simulink model "Squelette_DSPBuilder_FrameGenerator"  (R2016a)
settings: Solver=FixedStepDiscrete  StartTime=0.0  StopTime=2e-3  RelTol=1e-3
InitFcn:
  | %% DSPBuilder Start
  | alt_dspbuilder_update_model(bdroot)
  | %% DSPBuilder End
libraries: allblocks_alteradspbuilder2 x55
settings Model: Creator=rhev2401  LastModifiedBy=dufd2703
settings DataIOCC: LimitDataPoints=on  SaveFormat=Array  SignalLoggingSaveFormat=ModelDataLogs
settings DebuggingCC: SolverPrmCheckMsg=warning  MultiTaskDSMMsg=warning  MultiTaskCondExecSysMsg=none
settings HardwareCC: ProdBitPerPointer=32  ProdLargestAtomicFloat=None  ProdIntDivRoundTo=Undefined  ProdEndianess=Unspecified  ProdWordSize=32  ProdHWDeviceType=32-bit Generic
settings ModelReferenceCC: PropagateSignalLabelsOutOfModel=off
settings ConfigComp: CovModelRefEnable=Off  CovSFcnEnable=off

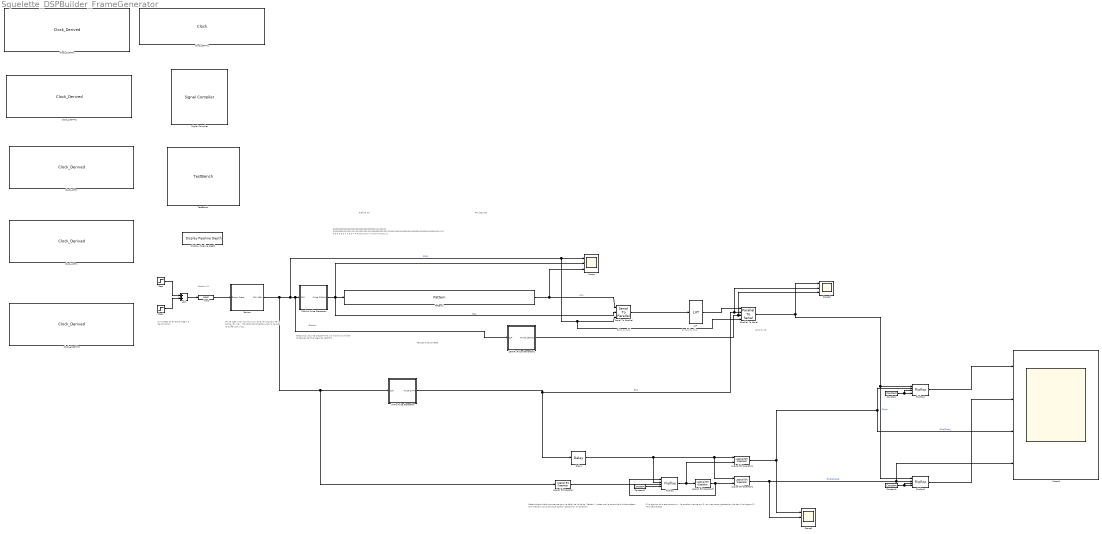
== system Squelette_DSPBuilder_FrameGenerator ==
  note: Simulates an event to begin a transmission
  note: Payload 80
  note: Prefixe 40
  note: 0000000000000000000000000000000011100101 10010000111011111111001101110100000101101110010100110001010100001010000110000110
      | 0 0 0 0 0 0 0 0 7 A 9 0 7 F F C E 2 8 6 7 A C 8 A 0 5 8 1 6
  note: Bouton 01
  note: On se crée une impulsion qui dure la longueur de la trame.
      |
      | En vrai, il faudrait transmettre jusqu'à ce que le buffer soit vide...
  note: Paquet à transmettre
  note: Bitclock
  note: Notez que, pour ce programme, on a choisi d'utiliser la fréquence d'horloge de 100MHz.
  note: Bit to symbol
  note: Symbol to chip
  note: Chip to I/Q
  note: Si le dernier chip est rentré sur I, le prochain rentre sur Q, et vice-versa; génération de deux horloges d'1 MHz déphasées
  note: Cette boîte à délai compense pour le délai de la boîte "Pattern" (notez que la sortie de la boîte pattern commence 1 coup de clock après l'apparition du Enable)
  250kHz Pulse Generator : Subsystem
  250kHz Pulse Generator1 : Subsystem
  2MHz Pulse Generator : Subsystem
  Add : Sum
  Bouton : Subsystem
  Clock_100MHz : allblocks_alteradspbuilder2/Clock_Derived  ClockNumerator=1  ClockDenominator=2  ResetLatency=0  ResetRegisterCascadeDepth=0  SimulationStartCycle=5  PhaseOffset=0  Reset=aclr_100MHz  ResetType=Active Low  Export=off
  Clock_125MHz : allblocks_alteradspbuilder2/Clock_Derived  ClockNumerator=10  ClockDenominator=25  ResetLatency=0  ResetRegisterCascadeDepth=0  SimulationStartCycle=5  PhaseOffset=0  Reset=aclr_125MHz  ResetType=Active Low  Export=off
  Clock_1MHz : allblocks_alteradspbuilder2/Clock_Derived  ClockNumerator=50  ClockDenominator=1  ResetLatency=0  ResetRegisterCascadeDepth=0  SimulationStartCycle=5  PhaseOffset=0  Reset=aclr_1MHz  ResetType=Active Low  Export=off
  Clock_2MHz : allblocks_alteradspbuilder2/Clock_Derived  ClockNumerator=25  ClockDenominator=1  ResetLatency=0  ResetRegisterCascadeDepth=0  SimulationStartCycle=5  PhaseOffset=0  Reset=aclr_2MHz  ResetType=Active Low  Export=off
  Clock_50MHz : allblocks_alteradspbuilder2/Clock  ClockPeriod=20  ClockPeriodUnit=ns  SampleTime=20e-9  ResetLatency=0  ResetRegisterCascadeDepth=0  SimulationStartCycle=5  PhaseOffset=0  Reset=aclr  ResetType=Active Low  Export=off
  Clock_62p5MHz : allblocks_alteradspbuilder2/Clock_Derived  ClockNumerator=800  ClockDenominator=1  ResetLatency=0  ResetRegisterCascadeDepth=0  SimulationStartCycle=5  PhaseOffset=0  Reset=aclr_62p5MHz  ResetType=Active Low  Export=off
  Constant : allblocks_alteradspbuilder2/Constant  mask_cst=1  BusType=Signed Integer  bwl=8  bwr=0  roundMode=Truncate  satMode=Wrap  SpecifyClock=off  allowFloatingPointOverride=on  logOutputs=off  logFile=U:\projet-s6\DSP builder\Squelette_FrameGenerator\tb_Squelette_DSPBuilder_FrameGenerator\Squelette%5FDSPBuilder%5FFrameGenerator_Constant.fixedpointlog
  Constant1 : allblocks_alteradspbuilder2/Constant  mask_cst=1  BusType=Signed Integer  bwl=8  bwr=0  roundMode=Truncate  satMode=Wrap  SpecifyClock=off  allowFloatingPointOverride=on  logOutputs=off  logFile=U:\projet-s6\DSP builder\Squelette_FrameGenerator\tb_Squelette_DSPBuilder_FrameGenerator\Squelette%5FDSPBuilder%5FFrameGenerator_Constant1.fixedpointlog
  Constant2 : allblocks_alteradspbuilder2/Constant  mask_cst=1  BusType=Signed Integer  bwl=8  bwr=0  roundMode=Truncate  satMode=Wrap  SpecifyClock=off  allowFloatingPointOverride=on  logOutputs=off  logFile=U:\projet-s6\DSP builder\Squelette_FrameGenerator\tb_Squelette_DSPBuilder_FrameGenerator\Squelette%5FDSPBuilder%5FFrameGenerator_Constant2.fixedpointlog
  Delay : allblocks_alteradspbuilder2/Delay  pipeline=1  pipeline_display=1  ClockPhase=1  use_ena=off  use_sclr=off  allowFloatingPointOverride=on  logOutputs=off  logFile=U:\projet-s6\DSP builder\Squelette_FrameGenerator\tb_Squelette_DSPBuilder_FrameGenerator\Squelette%5FDSPBuilder%5FFrameGenerator_Delay.fixedpointlog  use_init=off  reset_value=1
  Display Pipeline Depth : allblocks_alteradspbuilder2/Display Pipeline Depth  DisplayLatencyOnBlocks=on
  Flipflop : allblocks_alteradspbuilder2/Flipflop  mode=DFFE  BusType=Single Bit  bwl=2  bwr=2  pipeline_display=1
  Flipflop1 : allblocks_alteradspbuilder2/Flipflop  mode=DFFE  BusType=Single Bit  bwl=2  bwr=2  pipeline_display=1
  Flipflop2 : allblocks_alteradspbuilder2/Flipflop  mode=DFFE  BusType=Single Bit  bwl=2  bwr=2  pipeline_display=1
  Input : allblocks_alteradspbuilder2/Input  iofile=U:\projet-s6\DSP builder\Squelette_FrameGenerator\tb_Squelette_DSPBuilder_FrameGenerator\Squelette%5FDSPBuilder%5FFrameGenerator_Input.salt  BusType=Single Bit  bwl=1  bwr=0  SpecifyClock=on  clock=Clock_100MHz  PORTTYPE=Input  externalType=Inferred  allowFloatingPointOverride=on  logOutputs=off
  LUT : allblocks_alteradspbuilder2/LUT  addr_width=4  BusType=Unsigned Integer  bwl=32  bwr=0  init_array=chips_lut  allowFloatingPointOverride=on  logOutputs=off  logFile=U:\projet-s6\DSP builder\Squelette_FrameGenerator\tb_Squelette_DSPBuilder_FrameGenerator\Squelette%5FDSPBuilder%5FFrameGenerator_LUT.fixedpointlog  use_ena=off  reg_data=off  use_lpm=on  reg_addr=on  ram_type=AUTO  pipeline_display=1
  Logical Bit Operator : allblocks_alteradspbuilder2/Logical Bit Operator  LogicalOperator=NOT  user_inputs=2  pipeline_display=0
  Logical Bit Operator1 : allblocks_alteradspbuilder2/Logical Bit Operator  LogicalOperator=AND  user_inputs=2  pipeline_display=0
  Logical Bit Operator2 : allblocks_alteradspbuilder2/Logical Bit Operator  LogicalOperator=AND  user_inputs=2  pipeline_display=0
  Logical Bit Operator3 : allblocks_alteradspbuilder2/Logical Bit Operator  LogicalOperator=NOT  user_inputs=2  pipeline_display=0
  Parallel To Serial : allblocks_alteradspbuilder2/Parallel To Serial  BusType=Unsigned Integer  bwl=32  bwr=0  msbfirsttext=MSB First  msbfirst=1  repeatlastbit=off  use_ena=on  use_sclr=on
  Pattern1 : allblocks_alteradspbuilder2/Pattern  Sequence=<binary blob, 120 chars, not shown>  SpecifyClock=off  clock=Clock_250kHz  use_ena=on  use_sclr=off
  Scope : Scope  NumInputPorts=3
  Scope1 : Scope  NumInputPorts=4
  Scope2 : Scope  NumInputPorts=3
  Scope3 : Scope  NumInputPorts=3
  Serial To Parallel : allblocks_alteradspbuilder2/Serial To Parallel  BusType=Unsigned Integer  bwl=4  bwr=0  msbfirsttext=MSB First  msbfirst=1  use_ena=on  use_sclr=on
  Signal Compiler : allblocks_alteradspbuilder2/Signal Compiler  DeviceFamily=Cyclone V  DeviceName=AUTO  DisableEarlyHDLGeneration=off  EnableSignalTap=off  SignalTapDepth=128  UseBoardBlock=off  StpUseDefaultClock=on  StpClock=Clock_50MHz  ExportDir=C:\Users\pivd2501\Documents  MAX10_ProgrammingMode=Internal Flash (SDM) Single Boot
  Step : Step  Time=100e-6  Before=1  After=0  SampleTime=1/100e06  VectorParams1D=off
  Step1 : Step  Time=200e-6  SampleTime=1/100e06  VectorParams1D=off
  TestBench : allblocks_alteradspbuilder2/TestBench  enable=on  advancedMode=on  modelSimGui=on  maxDisplayErrors=1000  mismatchErrorLevel=Error  simdatafile=U:\projet-s6\DSP builder\Squelette_FrameGenerator\tb_Squelette_DSPBuilder_FrameGenerator\Squelette_DSPBuilder_FrameGenerator.simdata.tcl
  wires:
  Add/1 -> Input/1
  Step1/1 -> Add/2
  Step/1 -> Add/1
  250kHz Pulse Generator/1(Pulse 250kHz) -> Serial To Parallel/2, Pattern1/1, Scope/2  "ENA"
  Pattern1/1 -> Serial To Parallel/1, Scope/3  "ATA"
  Input/1 -> Bouton/1(Button Press)
  Serial To Parallel/1 -> LUT/1
  LUT/1 -> Parallel To Serial/1
  2MHz Pulse Generator/1(Pulse 2MHz) -> Scope3/2, Parallel To Serial/2, Delay/1  "ENA"
  Parallel To Serial/1 -> Flipflop1/1, Flipflop2/1, Scope3/1  "Chips"
  Bouton/1(CLR 480u) -> Logical Bit Operator/1, 2MHz Pulse Generator/1(CLR), 250kHz Pulse Generator1/1(CLR), 250kHz Pulse Generator/1(CLR), Parallel To Serial/4, Serial To Parallel/3, Scope/1  "SCLR"
  Flipflop/1 -> Logical Bit Operator1/2, Logical Bit Operator3/1
  Logical Bit Operator3/1 -> Flipflop/1, Logical Bit Operator2/2
  Logical Bit Operator1/1 -> Scope2/1, Scope1/3, Flipflop1/2  "ChipClock_I"
  Constant/1 -> Flipflop1/4, Flipflop1/3
  Constant1/1 -> Flipflop2/3, Flipflop2/4
  Logical Bit Operator2/1 -> Scope2/2, Scope1/4, Flipflop2/2  "ChipClock_Q"
  Logical Bit Operator/1 -> Flipflop/3
  Constant2/1 -> Flipflop/4
  Delay/1 -> Flipflop/2, Logical Bit Operator2/1, Logical Bit Operator1/1
  Flipflop2/1 -> Scope1/2
  Flipflop1/1 -> Scope1/1
  250kHz Pulse Generator1/1(Pulse 250kHz) -> Scope3/3, Parallel To Serial/3

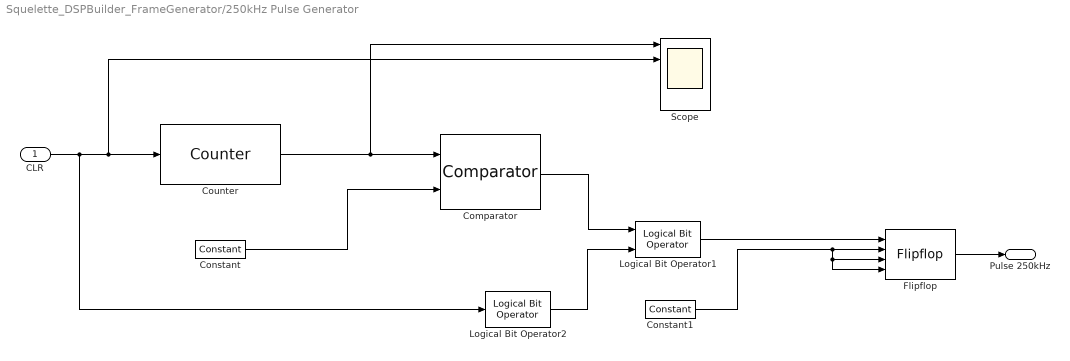
== system Squelette_DSPBuilder_FrameGenerator/250kHz Pulse Generator ==
  CLR : Inport
  Comparator : allblocks_alteradspbuilder2/Comparator  direction=a == b  pipeline_display=0  allowFloatingPointOverride=on  logOutputs=off  logFile=U:\projet-s6\DSP builder\Squelette_FrameGenerator\tb_Squelette_DSPBuilder_FrameGenerator\Squelette%5FDSPBuilder%5FFrameGenerator_250kHz+Pulse+Generator_Comparator.fixedpointlog
  Constant : allblocks_alteradspbuilder2/Constant  mask_cst=0  BusType=Unsigned Integer  bwl=1  bwr=0  roundMode=Truncate  satMode=Wrap  SpecifyClock=off  allowFloatingPointOverride=on  logOutputs=off  logFile=U:\projet-s6\DSP builder\Squelette_FrameGenerator\tb_Squelette_DSPBuilder_FrameGenerator\Squelette%5FDSPBuilder%5FFrameGenerator_250kHz+Pulse+Generator_Constant.fixedpointlog
  Constant1 : allblocks_alteradspbuilder2/Constant  mask_cst=1  BusType=Unsigned Integer  bwl=1  bwr=0  roundMode=Truncate  satMode=Wrap  SpecifyClock=off  allowFloatingPointOverride=on  logOutputs=off  logFile=U:\projet-s6\DSP builder\Squelette_FrameGenerator\tb_Squelette_DSPBuilder_FrameGenerator\Squelette%5FDSPBuilder%5FFrameGenerator_250kHz+Pulse+Generator_Constant1.fixedpointlog
  Counter : allblocks_alteradspbuilder2/Counter  BusType=Unsigned Integer  bwl=10  bwr=0  use_modulo=on  modulo=400  SpecifyClock=off  direction=Increment  use_sload=off  use_sset=off  svalue=1  use_clk_ena=off  use_ena=off  use_sclr=on  pipeline_display=1
  Flipflop : allblocks_alteradspbuilder2/Flipflop  mode=DFFE  BusType=Single Bit  bwl=2  bwr=2  pipeline_display=1
  Logical Bit Operator1 : allblocks_alteradspbuilder2/Logical Bit Operator  LogicalOperator=AND  user_inputs=2  pipeline_display=0
  Logical Bit Operator2 : allblocks_alteradspbuilder2/Logical Bit Operator  LogicalOperator=NOT  user_inputs=2  pipeline_display=0
  Scope : Scope  NumInputPorts=5
  Pulse 250kHz : Outport
  wires:
  Counter/1 -> Scope/1, Comparator/1
  Constant/1 -> Comparator/2
  CLR/1 -> Logical Bit Operator2/1, Scope/2, Counter/1
  Logical Bit Operator2/1 -> Logical Bit Operator1/2
  Comparator/1 -> Logical Bit Operator1/1
  Flipflop/1 -> Pulse 250kHz/1
  Logical Bit Operator1/1 -> Flipflop/1
  Constant1/1 -> Flipflop/4, Flipflop/3, Flipflop/2

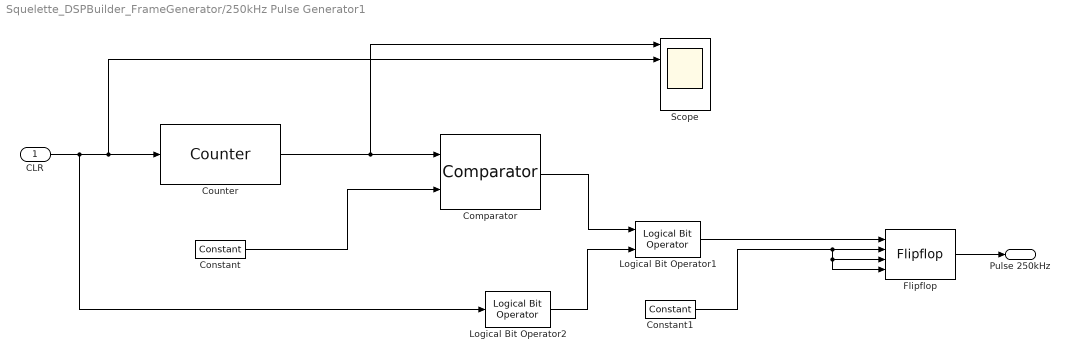
== system Squelette_DSPBuilder_FrameGenerator/250kHz Pulse Generator1 ==
  CLR : Inport
  Comparator : allblocks_alteradspbuilder2/Comparator  direction=a == b  pipeline_display=0  allowFloatingPointOverride=on  logOutputs=off  logFile=U:\projet-s6\DSP builder\Squelette_FrameGenerator\tb_Squelette_DSPBuilder_FrameGenerator\Squelette%5FDSPBuilder%5FFrameGenerator_250kHz+Pulse+Generator1_Comparator.fixedpointlog
  Constant : allblocks_alteradspbuilder2/Constant  mask_cst=0  BusType=Unsigned Integer  bwl=1  bwr=0  roundMode=Truncate  satMode=Wrap  SpecifyClock=off  allowFloatingPointOverride=on  logOutputs=off  logFile=U:\projet-s6\DSP builder\Squelette_FrameGenerator\tb_Squelette_DSPBuilder_FrameGenerator\Squelette%5FDSPBuilder%5FFrameGenerator_250kHz+Pulse+Generator1_Constant.fixedpointlog
  Constant1 : allblocks_alteradspbuilder2/Constant  mask_cst=1  BusType=Unsigned Integer  bwl=1  bwr=0  roundMode=Truncate  satMode=Wrap  SpecifyClock=off  allowFloatingPointOverride=on  logOutputs=off  logFile=U:\projet-s6\DSP builder\Squelette_FrameGenerator\tb_Squelette_DSPBuilder_FrameGenerator\Squelette%5FDSPBuilder%5FFrameGenerator_250kHz+Pulse+Generator1_Constant1.fixedpointlog
  Counter : allblocks_alteradspbuilder2/Counter  BusType=Unsigned Integer  bwl=12  bwr=0  use_modulo=on  modulo=1600  SpecifyClock=off  direction=Increment  use_sload=off  use_sset=off  svalue=1  use_clk_ena=off  use_ena=off  use_sclr=on  pipeline_display=1
  Flipflop : allblocks_alteradspbuilder2/Flipflop  mode=DFFE  BusType=Single Bit  bwl=2  bwr=2  pipeline_display=1
  Logical Bit Operator1 : allblocks_alteradspbuilder2/Logical Bit Operator  LogicalOperator=AND  user_inputs=2  pipeline_display=0
  Logical Bit Operator2 : allblocks_alteradspbuilder2/Logical Bit Operator  LogicalOperator=NOT  user_inputs=2  pipeline_display=0
  Scope : Scope  NumInputPorts=5
  Pulse 250kHz : Outport
  wires:
  Constant1/1 -> Flipflop/2, Flipflop/3, Flipflop/4
  Logical Bit Operator1/1 -> Flipflop/1
  Flipflop/1 -> Pulse 250kHz/1
  Comparator/1 -> Logical Bit Operator1/1
  Logical Bit Operator2/1 -> Logical Bit Operator1/2
  CLR/1 -> Counter/1, Scope/2, Logical Bit Operator2/1
  Constant/1 -> Comparator/2
  Counter/1 -> Comparator/1, Scope/1

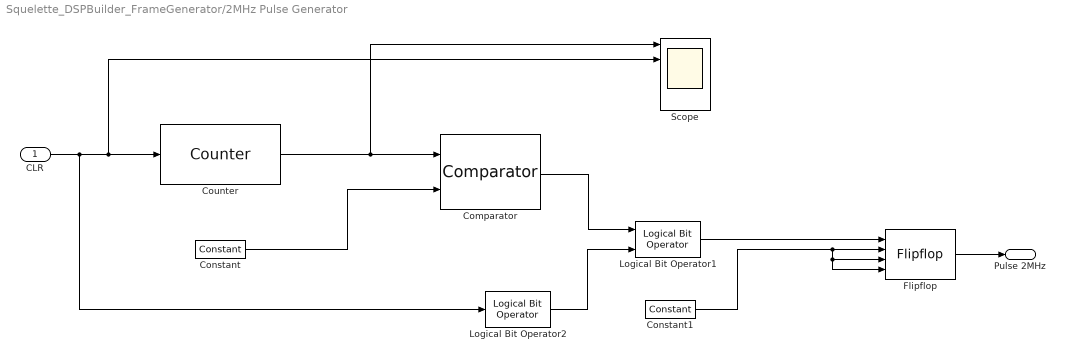
== system Squelette_DSPBuilder_FrameGenerator/2MHz Pulse Generator ==
  CLR : Inport
  Comparator : allblocks_alteradspbuilder2/Comparator  direction=a == b  pipeline_display=0  allowFloatingPointOverride=on  logOutputs=off  logFile=U:\projet-s6\DSP builder\Squelette_FrameGenerator\tb_Squelette_DSPBuilder_FrameGenerator\Squelette%5FDSPBuilder%5FFrameGenerator_2MHz+Pulse+Generator_Comparator.fixedpointlog
  Constant : allblocks_alteradspbuilder2/Constant  mask_cst=0  BusType=Unsigned Integer  bwl=1  bwr=0  roundMode=Truncate  satMode=Wrap  SpecifyClock=off  allowFloatingPointOverride=on  logOutputs=off  logFile=U:\projet-s6\DSP builder\Squelette_FrameGenerator\tb_Squelette_DSPBuilder_FrameGenerator\Squelette%5FDSPBuilder%5FFrameGenerator_2MHz+Pulse+Generator_Constant.fixedpointlog
  Constant1 : allblocks_alteradspbuilder2/Constant  mask_cst=1  BusType=Unsigned Integer  bwl=1  bwr=0  roundMode=Truncate  satMode=Wrap  SpecifyClock=off  allowFloatingPointOverride=on  logOutputs=off  logFile=U:\projet-s6\DSP builder\Squelette_FrameGenerator\tb_Squelette_DSPBuilder_FrameGenerator\Squelette%5FDSPBuilder%5FFrameGenerator_2MHz+Pulse+Generator_Constant1.fixedpointlog
  Counter : allblocks_alteradspbuilder2/Counter  BusType=Unsigned Integer  bwl=10  bwr=0  use_modulo=on  modulo=50  SpecifyClock=off  direction=Increment  use_sload=off  use_sset=off  svalue=1  use_clk_ena=off  use_ena=off  use_sclr=on  pipeline_display=1
  Flipflop : allblocks_alteradspbuilder2/Flipflop  mode=DFFE  BusType=Single Bit  bwl=2  bwr=2  pipeline_display=1
  Logical Bit Operator1 : allblocks_alteradspbuilder2/Logical Bit Operator  LogicalOperator=AND  user_inputs=2  pipeline_display=0
  Logical Bit Operator2 : allblocks_alteradspbuilder2/Logical Bit Operator  LogicalOperator=NOT  user_inputs=2  pipeline_display=0
  Scope : Scope  NumInputPorts=5
  Pulse 2MHz : Outport
  wires:
  Counter/1 -> Scope/1, Comparator/1
  Constant/1 -> Comparator/2
  CLR/1 -> Logical Bit Operator2/1, Scope/2, Counter/1
  Logical Bit Operator2/1 -> Logical Bit Operator1/2
  Comparator/1 -> Logical Bit Operator1/1
  Flipflop/1 -> Pulse 2MHz/1
  Logical Bit Operator1/1 -> Flipflop/1
  Constant1/1 -> Flipflop/4, Flipflop/3, Flipflop/2

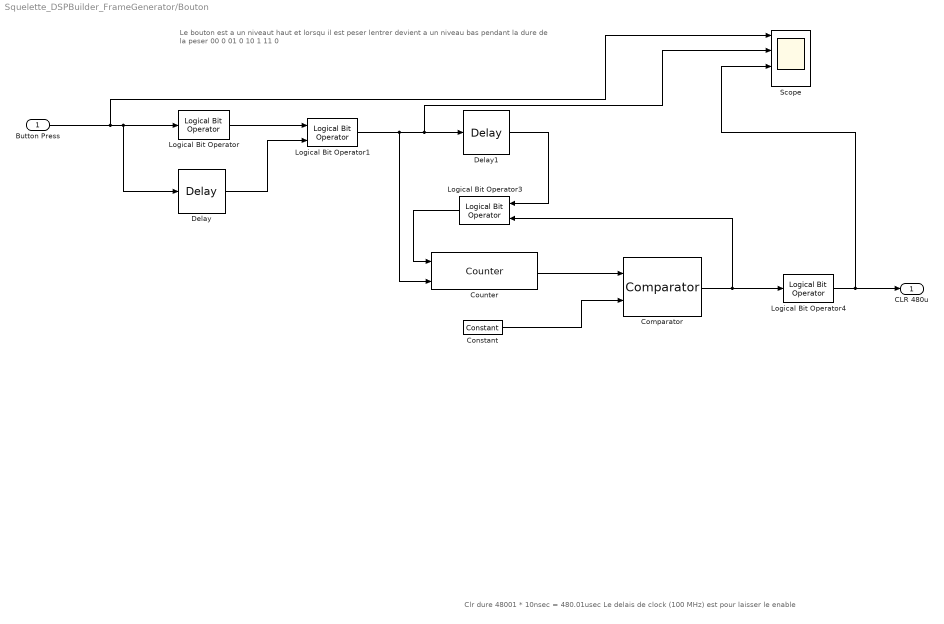
== system Squelette_DSPBuilder_FrameGenerator/Bouton ==
  note: Clr dure 48001 * 10nsec = 480.01usec Le delais de clock (100 MHz) est pour laisser le enable
  note: Le bouton est a un niveaut haut et lorsqu il est peser lentrer devient a un niveau bas pendant la dure de la peser
      |
      | 00  0
      | 01  0
      | 10  1
      | 11  0
  Button Press : Inport
  Comparator : allblocks_alteradspbuilder2/Comparator  direction=a >= b  pipeline_display=0  allowFloatingPointOverride=on  logOutputs=off  logFile=U:\projet-s6\DSP builder\Squelette_FrameGenerator\tb_Squelette_DSPBuilder_FrameGenerator\Squelette%5FDSPBuilder%5FFrameGenerator_Bouton_Comparator.fixedpointlog
  Constant : allblocks_alteradspbuilder2/Constant  mask_cst=1  BusType=Unsigned Integer  bwl=8  bwr=0  roundMode=Truncate  satMode=Wrap  SpecifyClock=off  allowFloatingPointOverride=on  logOutputs=off  logFile=U:\projet-s6\DSP builder\Squelette_FrameGenerator\tb_Squelette_DSPBuilder_FrameGenerator\Squelette%5FDSPBuilder%5FFrameGenerator_Bouton_Constant.fixedpointlog
  Counter : allblocks_alteradspbuilder2/Counter  BusType=Unsigned Integer  bwl=16  bwr=0  use_modulo=on  modulo=48001  SpecifyClock=off  clock=Clock_100MHz  direction=Increment  use_sload=off  use_sset=off  svalue=1  use_clk_ena=off  use_ena=on  use_sclr=on  pipeline_display=1
  Delay : allblocks_alteradspbuilder2/Delay  pipeline=1  pipeline_display=1  ClockPhase=1  use_ena=off  use_sclr=off  allowFloatingPointOverride=on  logOutputs=off  logFile=U:\projet-s6\DSP builder\Squelette_FrameGenerator\tb_Squelette_DSPBuilder_FrameGenerator\Squelette%5FDSPBuilder%5FFrameGenerator_Bouton_Delay.fixedpointlog  use_init=off  reset_value=1
  Delay1 : allblocks_alteradspbuilder2/Delay  pipeline=1  pipeline_display=1  ClockPhase=1  use_ena=off  use_sclr=off  allowFloatingPointOverride=on  logOutputs=off  logFile=U:\projet-s6\DSP builder\Squelette_FrameGenerator\tb_Squelette_DSPBuilder_FrameGenerator\Squelette%5FDSPBuilder%5FFrameGenerator_Bouton_Delay1.fixedpointlog  use_init=off  reset_value=1
  Logical Bit Operator : allblocks_alteradspbuilder2/Logical Bit Operator  LogicalOperator=NOT  user_inputs=2  pipeline_display=0
  Logical Bit Operator1 : allblocks_alteradspbuilder2/Logical Bit Operator  LogicalOperator=AND  user_inputs=2  pipeline_display=0
  Logical Bit Operator3 : allblocks_alteradspbuilder2/Logical Bit Operator  LogicalOperator=OR  user_inputs=2  pipeline_display=0
  Logical Bit Operator4 : allblocks_alteradspbuilder2/Logical Bit Operator  LogicalOperator=NOT  user_inputs=2  pipeline_display=0
  Scope : Scope  NumInputPorts=4
  CLR 480u : Outport
  wires:
  Button Press/1 -> Scope/1, Logical Bit Operator/1, Delay/1
  Logical Bit Operator/1 -> Logical Bit Operator1/1
  Logical Bit Operator1/1 -> Scope/2, Delay1/1, Counter/2
  Counter/1 -> Comparator/1
  Constant/1 -> Comparator/2
  Delay1/1 -> Logical Bit Operator3/1
  Logical Bit Operator3/1 -> Counter/1
  Comparator/1 -> Logical Bit Operator3/2, Logical Bit Operator4/1
  Delay/1 -> Logical Bit Operator1/2
  Logical Bit Operator4/1 -> Scope/3, CLR 480u/1
